simulink model "control2_mm"  (R2014b)
settings: Solver=ode45  StartTime=0.0  StopTime=20  RelTol=1e-3
undefined symbols (not defined in the file or in its folder): JacFinv2, posicionmm, trayectorias
libraries: simulink x3, LibrarySimulinkSAS x1
settings Model: Creator=Kelly  LastModifiedBy=heredia

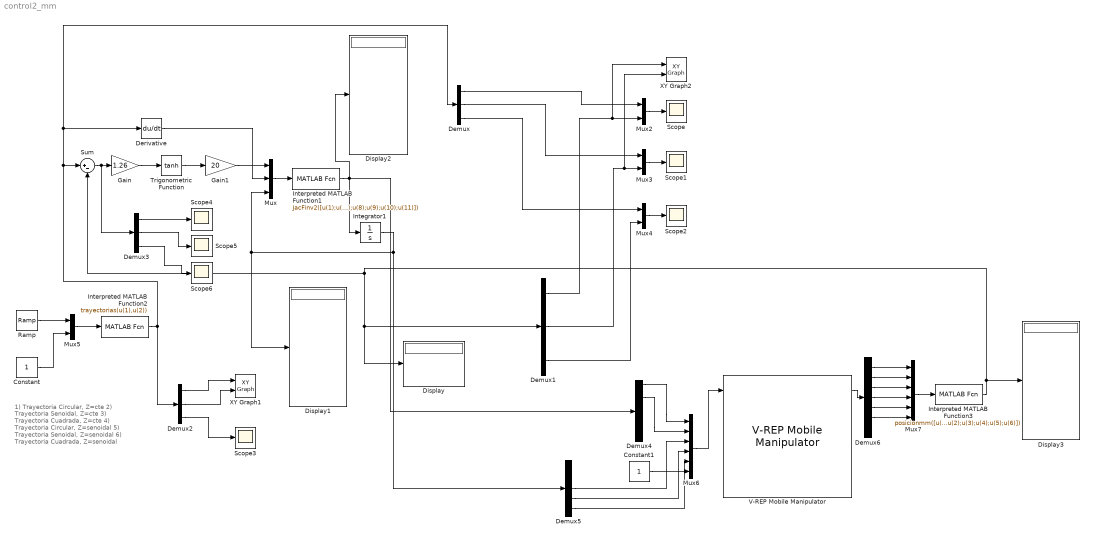
== system control2_mm ==
  note: 1) Trayectoria Circular, Z=cte
      | 2) Trayectoria Senoidal, Z=cte
      | 3) Trayectoria Cuadrada, Z=cte
      | 4) Trayectoria Circular, Z=senoidal
      | 5) Trayectoria Senoidal, Z=senoidal
      | 6) Trayectoria Cuadrada, Z=senoidal
  Constant : Constant
  Constant1 : Constant
  Demux{,1..3} (4 alike) : Demux  Outputs=3
  Demux4 : Demux  Outputs=5
  Demux5 : Demux  Outputs=5
  Demux6 : Demux  Outputs=7
  Derivative : Derivative
  Display{,1..3} (4 alike) : Display
  Gain : Gain  Gain=1.26
  Gain1 : Gain  Gain=20
  Integrator1 : Integrator  InitialCondition="[0 0 pi/2  0 0]"
  Interpreted MATLAB Function1 : MATLABFcn  MATLABFcn=JacFinv2([u(1);u(2);u(3)],[u(4);u(5);u(6)],[u(7);u(8);u(9);u(10);u(11)])
  Interpreted MATLAB Function2 : MATLABFcn  MATLABFcn=trayectorias(u(1),u(2))  OutputDimensions=3
  Interpreted MATLAB Function3 : MATLABFcn  MATLABFcn=posicionmm([u(1);u(2);u(3);u(4);u(5);u(6)])
  Mux : Mux  Inputs=3
  Mux{2..5} (4 alike) : Mux  Inputs=2
  Mux6 : Mux  Inputs=6
  Mux7 : Mux  Inputs=6
  Ramp : simulink/Sources/Ramp  slope=1  start=0  X0=0
  Scope{,1..6} (7 alike) : Scope
      Scope settings: YMin=1.5  YMax=4.5
      Scope1 settings: YMin=-1.5  YMax=1.5
      Scope2 settings: TimeRange=20  YMin=-0  YMax=2  SaveName=ScopeData2
      Scope3 settings: YMin=0  YMax=10  SaveName=ScopeData3
      Scope4 settings: YMin=0  YMax=0.0006  SaveName=ScopeData4
      Scope5 settings: YMin=-1e-32  YMax=3e-32  SaveName=ScopeData5
      Scope6 settings: YMin=-0.0004  YMax=0.0006  SaveName=ScopeData6
  Sum : Sum  Inputs=|+-
  Trigonometric Function : Trigonometry  Operator=tanh
  V-REP Mobile Manipulator : LibrarySimulinkSAS/V-REP Mobile Manipulator  id1=1  id2=2
  XY Graph1 : simulink/Sinks/XY Graph  xmin=2.5  xmax=8.5  ymin=-0.5  ymax=5.5  st=-1
  XY Graph2 : simulink/Sinks/XY Graph  xmin=2.5  xmax=8.5  ymin=-0.5  ymax=5.5  st=-1
  wires:
  Mux/1 -> Interpreted MATLAB Function1/1
  Interpreted MATLAB Function3/1 -> Display3/1, Display/1, Demux1/1, Sum/2
  Sum/1 -> Demux3/1, Gain/1
  Interpreted MATLAB Function2/1 -> Demux2/1, Sum/1, Derivative/1, Demux/1
  Integrator1/1 -> Demux5/1, Display1/1, Mux/3
  Mux4/1 -> Scope2/1
  Mux3/1 -> Scope1/1
  Mux2/1 -> Scope/1
  Demux/1 -> Mux2/1
  Demux/2 -> Mux3/1
  Demux/3 -> Mux4/1
  Trigonometric Function/1 -> Gain1/1
  Mux5/1 -> Interpreted MATLAB Function2/1
  Ramp/1 -> Mux5/1
  Constant/1 -> Mux5/2
  Demux1/2 -> XY Graph2/2, Mux3/2
  Demux1/3 -> Mux4/2
  Demux2/1 -> XY Graph1/1
  Demux2/2 -> XY Graph1/2
  Demux2/3 -> Scope3/1
  Gain/1 -> Trigonometric Function/1
  Gain1/1 -> Mux/1
  Derivative/1 -> Mux/2
  Demux1/1 -> XY Graph2/1, Mux2/2
  Demux3/1 -> Scope4/1
  Demux3/3 -> Scope6/1
  Demux3/2 -> Scope5/1
  Interpreted MATLAB Function1/1 -> Demux4/1, Display2/1, Integrator1/1
  Demux4/1 -> Mux6/1
  Demux4/2 -> Mux6/2
  Demux5/3 -> Mux6/3
  Demux5/4 -> Mux6/4
  Demux5/5 -> Mux6/5
  Mux6/1 -> V-REP Mobile Manipulator/1
  Constant1/1 -> Mux6/6
  V-REP Mobile Manipulator/1 -> Demux6/1
  Demux6/1 -> Mux7/1
  Demux6/2 -> Mux7/2
  Demux6/3 -> Mux7/3
  Demux6/4 -> Mux7/4
  Demux6/5 -> Mux7/5
  Demux6/6 -> Mux7/6
  Mux7/1 -> Interpreted MATLAB Function3/1
